simulink model "Gear_Ratio_Sizing_Two_Speed"  (R2021a)
settings: Solver=FixedStepAuto  StartTime=0.0  StopTime=1372  FixedStep=1  MaxStep=1  RelTol=1e-3
values from neighbouring files (symbols this model uses):
  Cd = 0.28    [Gear_Ratio_Sizing_Two_Speed_Transmission.m]    (also in Two_Speed_Transmission_Optimization.m)
  Crf = 0.015    [Gear_Ratio_Sizing_Two_Speed_Transmission.m]    (also in Two_Speed_Transmission_Optimization.m)
  Fa = 3.8056    [Gear_Ratio_Sizing_Two_Speed_Transmission.m]    (also in Two_Speed_Transmission_Optimization.m)
  G1 = G1_range(i,j)    [Two_Speed_Transmission_Optimization.m]
  G2 = G2_range(i,j)    [Two_Speed_Transmission_Optimization.m]
  GVM = Mv+Md    (= 1730.665)    [Gear_Ratio_Sizing_Two_Speed_Transmission.m]    (also in Two_Speed_Transmission_Optimization.m)
  GVW = GVM*g    (= 16977.82365)    [Gear_Ratio_Sizing_Two_Speed_Transmission.m]    (also in Two_Speed_Transmission_Optimization.m)
  MMeff = data(:,2:16)    [Gear_Ratio_Sizing_Two_Speed_Transmission.m]    (also in Two_Speed_Transmission_Optimization.m)
  MMeff_Speed = data(:,1)    [Gear_Ratio_Sizing_Two_Speed_Transmission.m]    (also in Two_Speed_Transmission_Optimization.m)
  MMeff_Torque = data(:,17)    [Gear_Ratio_Sizing_Two_Speed_Transmission.m]    (also in Two_Speed_Transmission_Optimization.m)
  rho = 1.225    [Gear_Ratio_Sizing_Two_Speed_Transmission.m]    (also in Two_Speed_Transmission_Optimization.m)
  Rw = 0.2032    [Gear_Ratio_Sizing_Two_Speed_Transmission.m]    (also in Two_Speed_Transmission_Optimization.m)
  Teff = 0.89    [Gear_Ratio_Sizing_Two_Speed_Transmission.m]    (also in Two_Speed_Transmission_Optimization.m)
  V_shift = 25    [Gear_Ratio_Sizing_Two_Speed_Transmission.m]    (also in Two_Speed_Transmission_Optimization.m)
settings Model: Creator=LENOVO  LastModifiedBy=LENOVO

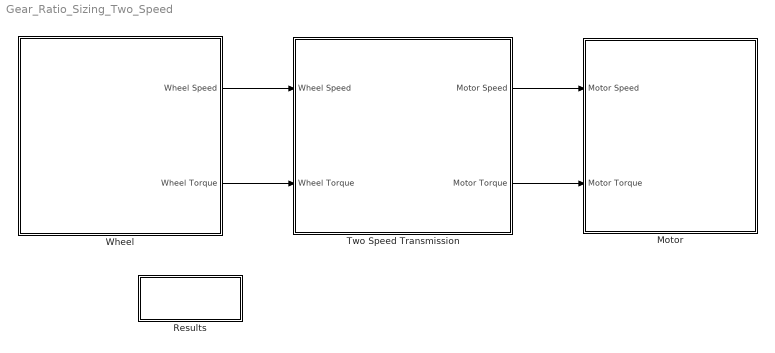
== system Gear_Ratio_Sizing_Two_Speed ==
  Motor : Subsystem
  Results : Subsystem
  Two Speed Transmission : Subsystem
  Wheel : Subsystem
  wires:
  Two Speed Transmission/2(Motor Torque) -> Motor/2(Motor Torque)
  Two Speed Transmission/1(Motor Speed) -> Motor/1(Motor Speed)
  Wheel/2(Wheel Torque) -> Two Speed Transmission/2(Wheel Torque)
  Wheel/1(Wheel Speed) -> Two Speed Transmission/1(Wheel Speed)

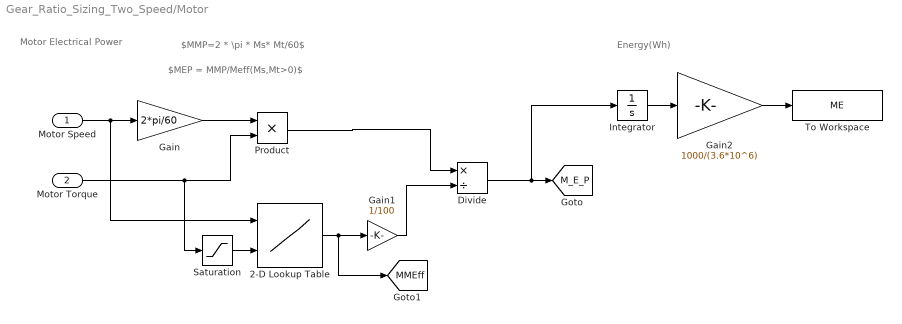
== system Gear_Ratio_Sizing_Two_Speed/Motor ==
  note: Energy(Wh)
  note: Motor Electrical Power
  note: $MEP = MMP/Meff(Ms,Mt>0)$
  note: $MMP=2 * \pi * Ms* Mt/60$
  Motor Speed : Inport
  Motor Torque : Inport  Port=2
  2-D Lookup Table : Lookup_n-D  BreakpointsForDimension1=MMeff_Speed  BreakpointsForDimension2=MMeff_Torque  Table=MMeff  InternalRulePriority=Speed  RndMeth=Simplest  InputSameDT=on
      settings: InputPortMap=u0,u1
  Divide : Product  Inputs=*/
  Gain : Gain  Gain=2*pi/60
  Gain1 : Gain  Gain=1/100
  Gain2 : Gain  Gain=1000/(3.6*10^6)
  Integrator : Integrator
  Product : Product
  Saturation : Saturate  UpperLimit=inf  LowerLimit=0
  To Workspace : ToWorkspace  VariableName=ME  SaveFormat=Timeseries  SampleTime=-1
  tag scope: MMEff=global, M_E_P=global
  wires:
  Gain/1 -> Product/1
  Motor Torque/1 -> Saturation/1, Product/2
  Product/1 -> Divide/1
  Motor Speed/1 -> 2-D Lookup Table/1, Gain/1
  Gain1/1 -> Divide/2
  Divide/1 -> Integrator/1, [M_E_P]
  2-D Lookup Table/1 -> [MMEff], Gain1/1
  Integrator/1 -> Gain2/1
  Gain2/1 -> To Workspace/1
  Saturation/1 -> 2-D Lookup Table/2

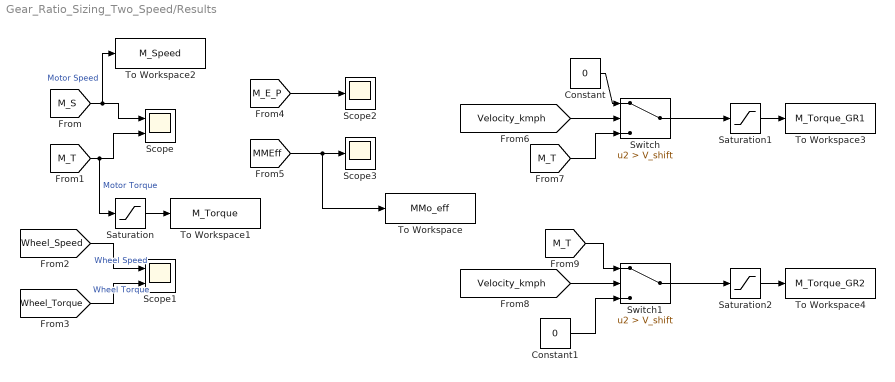
== system Gear_Ratio_Sizing_Two_Speed/Results ==
  Constant : Constant  Value=0
  Constant1 : Constant  Value=0
  Saturation : Saturate  UpperLimit=inf  LowerLimit=0
  Saturation1 : Saturate  UpperLimit=inf  LowerLimit=0
  Saturation2 : Saturate  UpperLimit=inf  LowerLimit=0
  Scope : Scope  NumInputPorts=2
  Scope1 : Scope  NumInputPorts=2
  Scope2 : Scope
  Scope3 : Scope
  Switch : Switch  Criteria=u2 > Threshold  Threshold=V_shift
  Switch1 : Switch  Criteria=u2 > Threshold  Threshold=V_shift
  To Workspace : ToWorkspace  VariableName=MMo_eff  SaveFormat=Timeseries  SampleTime=-1
  To Workspace1 : ToWorkspace  VariableName=M_Torque  SaveFormat=Timeseries  SampleTime=-1
  To Workspace2 : ToWorkspace  VariableName=M_Speed  SaveFormat=Timeseries  SampleTime=-1
  To Workspace3 : ToWorkspace  VariableName=M_Torque_GR1  SaveFormat=Timeseries  SampleTime=-1
  To Workspace4 : ToWorkspace  VariableName=M_Torque_GR2  SaveFormat=Timeseries  SampleTime=-1
  wires:
  [M_S] -> To Workspace2/1, Scope/1  "Motor Speed"
  [M_T] -> Saturation/1, Scope/2  "Motor Torque"
  [Wheel_Speed] -> Scope1/1  "Wheel Speed"
  [Wheel_Torque] -> Scope1/2  "Wheel Torque"
  [M_E_P] -> Scope2/1
  [MMEff] -> To Workspace/1, Scope3/1
  Saturation/1 -> To Workspace1/1
  Saturation1/1 -> To Workspace3/1
  Switch/1 -> Saturation1/1
  [Velocity_kmph] -> Switch/2
  [M_T] -> Switch/3
  Constant/1 -> Switch/1
  Switch1/1 -> Saturation2/1
  Saturation2/1 -> To Workspace4/1
  [Velocity_kmph] -> Switch1/2
  Constant1/1 -> Switch1/3
  [M_T] -> Switch1/1

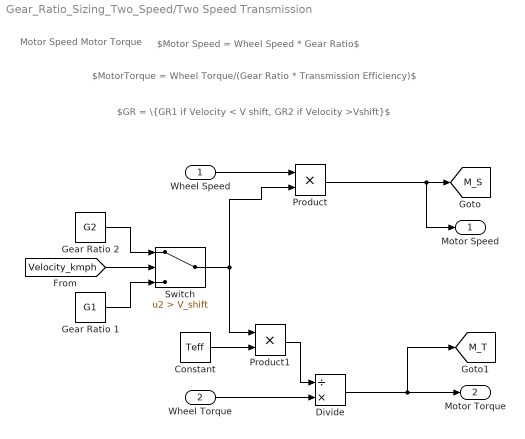
== system Gear_Ratio_Sizing_Two_Speed/Two Speed Transmission ==
  note: $GR = \{GR1 if Velocity < V shift, GR2 if Velocity >Vshift}$
  note: Motor Speed
      | Motor Torque
  note: $MotorTorque = Wheel Torque/(Gear Ratio * Transmission Efficiency)$
  note: $Motor Speed = Wheel Speed * Gear Ratio$
  Wheel Speed : Inport
  Wheel Torque : Inport  Port=2
  Constant : Constant  Value=Teff
  Divide : Product  Inputs=/*
  Gear Ratio 1 : Constant  Value=G1
  Gear Ratio 2 : Constant  Value=G2
  Product : Product
  Product1 : Product
  Switch : Switch  Criteria=u2 > Threshold  Threshold=V_shift
  Motor Speed : Outport
  Motor Torque : Outport  Port=2
  tag scope: M_S=global, M_T=global
  wires:
  Wheel Torque/1 -> Divide/2
  Divide/1 -> [M_T], Motor Torque/1
  Product1/1 -> Divide/1
  Constant/1 -> Product1/2
  Wheel Speed/1 -> Product/1
  Product/1 -> Motor Speed/1, [M_S]
  [Velocity_kmph] -> Switch/2
  Gear Ratio 2/1 -> Switch/1
  Gear Ratio 1/1 -> Switch/3
  Switch/1 -> Product1/1, Product/2

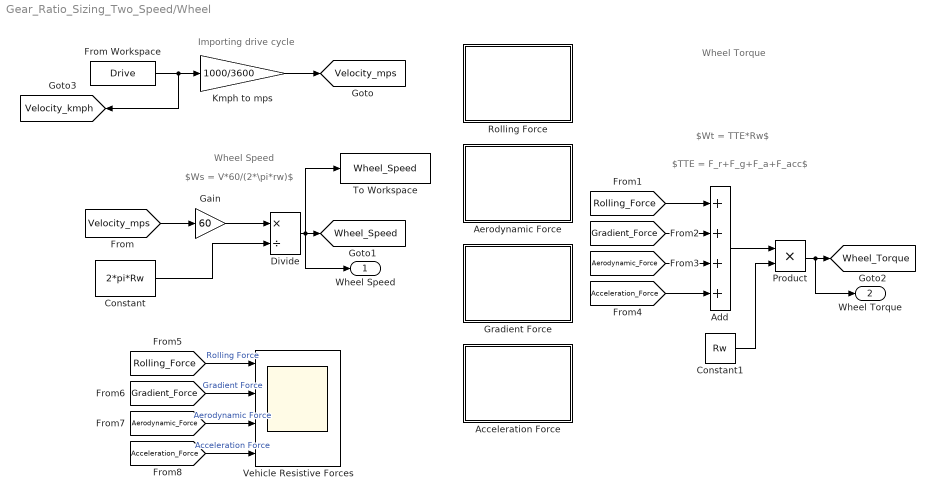
== system Gear_Ratio_Sizing_Two_Speed/Wheel ==
  note: $TTE = F_r+F_g+F_a+F_acc$
  note: $Wt = TTE*Rw$
  note: Wheel Torque
  note: $Ws = V*60/(2*\pi*rw)$
  note: Wheel Speed
  note: Importing drive cycle
  Acceleration Force : Subsystem
  Add : Sum  Inputs=4
  Aerodynamic Force : Subsystem
  Constant : Constant  Value=2*pi*Rw
  Constant1 : Constant  Value=Rw
  Divide : Product  Inputs=*/
  From Workspace : FromWorkspace  VariableName=Drive
  Gain : Gain  Gain=60
  Gradient Force : Subsystem
  Kmph to mps : Gain  Gain=1000/3600
  Product : Product
  Rolling Force : Subsystem
  To Workspace : ToWorkspace  VariableName=Wheel_Speed  SaveFormat=Timeseries  SampleTime=-1
  Vehicle Resistive Forces : Scope  NumInputPorts=4
  Wheel Speed : Outport
  Wheel Torque : Outport  Port=2
  tag scope: Velocity_kmph=global, Velocity_mps=global, Wheel_Speed=global, Wheel_Torque=global
  wires:
  From Workspace/1 -> [Velocity_kmph], Kmph to mps/1
  Kmph to mps/1 -> [Velocity_mps]
  [Velocity_mps] -> Gain/1
  Gain/1 -> Divide/1
  Constant/1 -> Divide/2
  Divide/1 -> To Workspace/1, [Wheel_Speed], Wheel Speed/1
  [Rolling_Force] -> Add/1
  [Gradient_Force] -> Add/2
  [Aerodynamic_Force] -> Add/3
  [Acceleration_Force] -> Add/4
  Add/1 -> Product/1
  Constant1/1 -> Product/2
  Product/1 -> Wheel Torque/1, [Wheel_Torque]
  [Rolling_Force] -> Vehicle Resistive Forces/1  "Rolling Force"
  [Gradient_Force] -> Vehicle Resistive Forces/2  "Gradient Force"
  [Aerodynamic_Force] -> Vehicle Resistive Forces/3  "Aerodynamic Force"
  [Acceleration_Force] -> Vehicle Resistive Forces/4  "Acceleration Force"

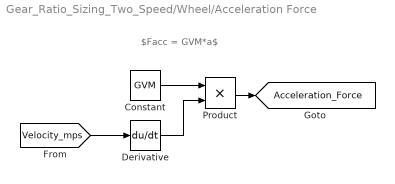
== system Gear_Ratio_Sizing_Two_Speed/Wheel/Acceleration Force ==
  note: $Facc = GVM*a$
  Constant : Constant  Value=GVM
  Derivative : Derivative
  Product : Product
  tag scope: Acceleration_Force=global
  wires:
  [Velocity_mps] -> Derivative/1
  Constant/1 -> Product/1
  Derivative/1 -> Product/2
  Product/1 -> [Acceleration_Force]

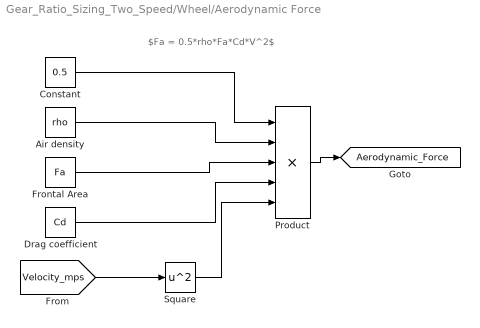
== system Gear_Ratio_Sizing_Two_Speed/Wheel/Aerodynamic Force ==
  note: $Fa = 0.5*rho*Fa*Cd*V^2$
  Air density : Constant  Value=rho
  Constant : Constant  Value=0.5
  Drag coefficient : Constant  Value=Cd
  Frontal Area : Constant  Value=Fa
  Product : Product  Inputs=5
  Square : Math  Operator=square  SaturateOnIntegerOverflow=on
  tag scope: Aerodynamic_Force=global
  wires:
  [Velocity_mps] -> Square/1
  Square/1 -> Product/5
  Drag coefficient/1 -> Product/4
  Frontal Area/1 -> Product/3
  Air density/1 -> Product/2
  Constant/1 -> Product/1
  Product/1 -> [Aerodynamic_Force]

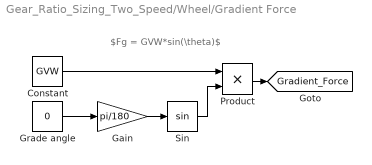
== system Gear_Ratio_Sizing_Two_Speed/Wheel/Gradient Force ==
  note: $Fg = GVW*sin(\theta)$
  Constant : Constant  Value=GVW
  Gain : Gain  Gain=pi/180
  Grade angle : Constant  Value=0
  Product : Product
  Sin : Trigonometry
  tag scope: Gradient_Force=global
  wires:
  Grade angle/1 -> Gain/1
  Gain/1 -> Sin/1
  Constant/1 -> Product/1
  Sin/1 -> Product/2
  Product/1 -> [Gradient_Force]

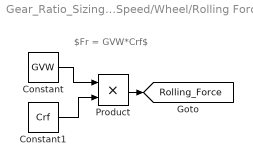
== system Gear_Ratio_Sizing_Two_Speed/Wheel/Rolling Force ==
  note: $Fr = GVW*Crf$
  Constant : Constant  Value=GVW
  Constant1 : Constant  Value=Crf
  Product : Product
  tag scope: Rolling_Force=global
  wires:
  Constant/1 -> Product/1
  Constant1/1 -> Product/2
  Product/1 -> [Rolling_Force]
